simulink model "H_inf_sim"  (R2022b)
settings: Solver=VariableStepAuto  StartTime=0.0  StopTime=10  RelTol=1e-3
values from neighbouring files (symbols this model uses):
  A = [-0.051 0 -0.144 -0.056 0 0 0 0 0 0 0 0 ... (169 elements, 13x13)]    [Elicottero.mat]
  B = [0 0 0 0 0 0 0.68 3.043 0 0 0 0 ... (52 elements, 13x4)]    [Elicottero.mat]
undefined symbols (not defined in the file or in its folder): C, D
libraries: cstblocks x3
settings Model: Creator=valen  LastModifiedBy=valen
settings ModelReferenceCC: EnableRefExpFcnMdlSchedulingChecks=on

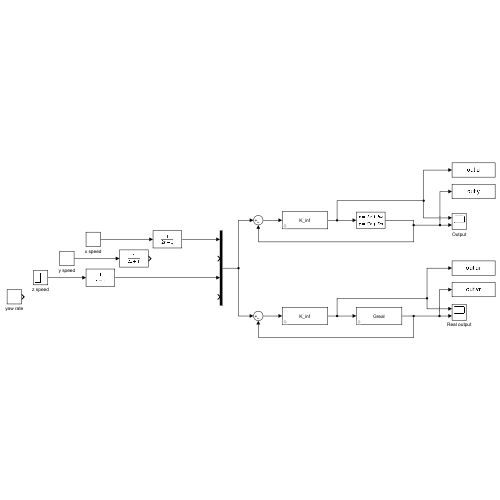
[thumbnail: Simulink's stored preview of the top-level diagram]
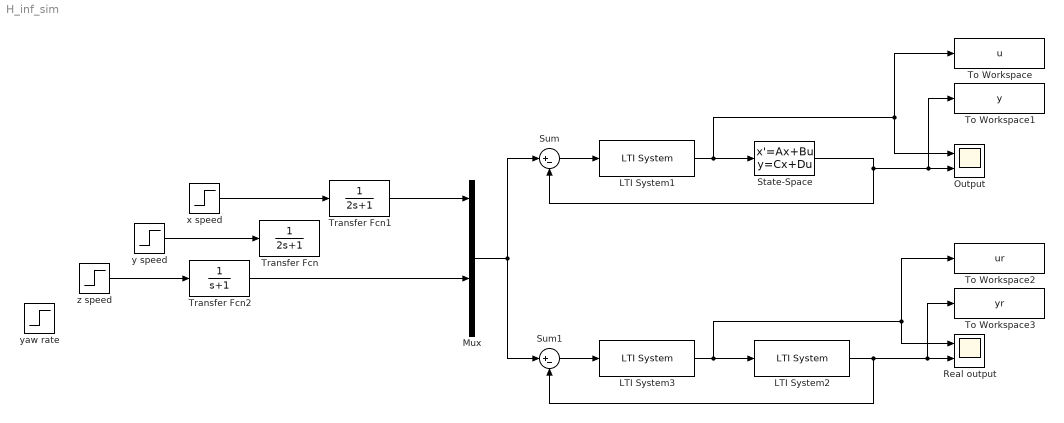
== system H_inf_sim ==
  LTI System1 : cstblocks/LTI System  sys=K_inf  IC=[]
  LTI System2 : cstblocks/LTI System  sys=Greal  IC=[]
  LTI System3 : cstblocks/LTI System  sys=K_inf  IC=[]
  Mux : Mux
  Output : Scope  NumInputPorts=2
  Real output : Scope  NumInputPorts=2
  State-Space : StateSpace  A=A  B=B  C=C  D=D  InitialCondition=0
  Sum : Sum  Inputs=|+-
  Sum1 : Sum  Inputs=|+-
  To Workspace : ToWorkspace  VariableName=u  SaveFormat=Structure With Time  SampleTime=-1
  To Workspace1 : ToWorkspace  VariableName=y  SaveFormat=Structure With Time  SampleTime=-1
  To Workspace2 : ToWorkspace  VariableName=ur  SaveFormat=Structure With Time  SampleTime=-1
  To Workspace3 : ToWorkspace  VariableName=yr  SaveFormat=Structure With Time  SampleTime=-1
  Transfer Fcn : TransferFcn  Denominator=[2 1]
  Transfer Fcn1 : TransferFcn  Denominator=[2 1]
  Transfer Fcn2 : TransferFcn  Denominator=[1 1]
  x speed : Step  Time=0  SampleTime=0
  y speed : Step  Time=0  SampleTime=0
  yaw rate : Step  Time=0  SampleTime=0
  z speed : Step  Time=3  After=0.5  SampleTime=0
  wires:
  LTI System1/1 -> To Workspace/1, Output/1, State-Space/1
  Sum/1 -> LTI System1/1
  State-Space/1 -> Sum/2, To Workspace1/1, Output/2
  LTI System2/1 -> To Workspace3/1, Real output/2, Sum1/2
  Sum1/1 -> LTI System3/1
  LTI System3/1 -> Real output/1, To Workspace2/1, LTI System2/1
  Mux/1 -> Sum1/1, Sum/1
  y speed/1 -> Transfer Fcn/1
  x speed/1 -> Transfer Fcn1/1
  z speed/1 -> Transfer Fcn2/1
  Transfer Fcn1/1 -> Mux/1
  Transfer Fcn2/1 -> Mux/3
